simulink model "rlsest"  (Simulink 6.0)
settings: Solver=VariableStepDiscrete  SolverMode=SingleTasking  StartTime=0.0  StopTime=200  MaxStep=1  RelTol=1e-3  AbsTol=1e-6
StartFcn:
  | rlspps([],[],[],'reset',find_system(get_param(gcs,'Handle'),'LookUnderMasks','all','Tag','PPC'));
settings Model: Creator=The MathWorks Inc.  LastModifiedBy=batserve  ExtModeTrigMode=oneshot  ExtModeArmWhenConnect=off  ExtModeAutoUpdateStatusClock=off
settings DataIOCC: ExternalInput=[]  LimitDataPoints=off  SaveOutput=off  SaveTime=off
settings OptimizationCC: BooleanDataType=off
settings DebuggingCC: CheckExecutionContextPreStartOutputMsg=on  CheckExecutionContextRuntimeOutputMsg=on  SolverPrmCheckMsg=none  IntegerOverflowMsg=none
settings HardwareCC: TargetUnknown=on

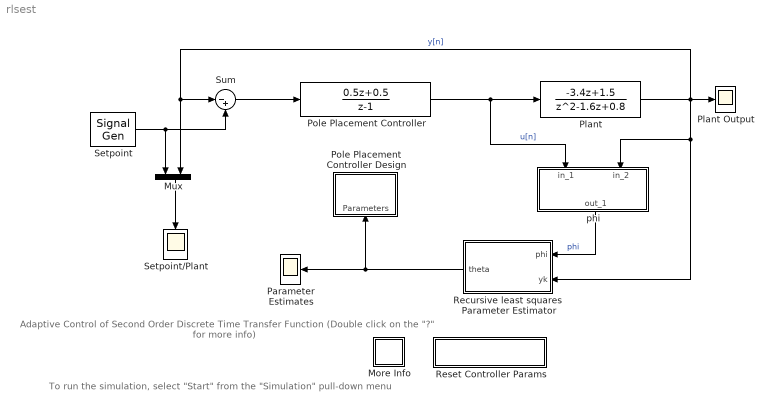
== system rlsest ==
  note: Adaptive Control of Second Order
      | Discrete Time Transfer Function
      | (Double click on the "?" for more info)
  note: To run the simulation, select "Start"
      | from the "Simulation" pull-down menu
  More Info : Subsystem  PropExecContextAcrossSSBoundary=on
      mask Display: disp('?')
  Mux : Mux  Orientation=down  Inputs=2
  Parameter Estimates : Scope
      settings: TickLabels=on  TimeRange=100.000000  DataFormat=Array
  Plant : DiscreteTransferFcn  Numerator=[-3.4 1.5]  Denominator=[1 -1.6 0.8]
  Plant Output : Scope
      settings: TickLabels=on  TimeRange=100.000000  DataFormat=Array
  Pole Placement Controller Design : Subsystem  Orientation=up  PropExecContextAcrossSSBoundary=on  mask(Pole Placement){@1=rlsest/Pole Placement Controller, @2=2, @3=poly([.6 .6 .6]), @4=10}
      mask prompts: @1 "Block name:"; @2 "Model order:"; @3 "Characteristic polynomial:"; @4 "Sample time:"
      mask help: Pole placement controller - installs new controller gains based upon a characteristic polynomial.
      mask init:
      | name=&1;order=@2;char_poly=@3;ts=@4;
      mask Help: Implements a pole placement design scheme for a discrete time controller.  Change the characteristic polynomial to see how the closed loop behavior changes.
      mask Display: disp('rlsppd')
  Pole Placement Controller : DiscreteTransferFcn  Tag=PPC  Numerator=[0.5 0.5]  Denominator=[1 -1]
  Recursive least squares  Parameter Estimator : Subsystem  Orientation=left  PropExecContextAcrossSSBoundary=on  mask(RLS Estimator){@1=2, @2=0.8, @3=1}
      mask prompts: @1 "Model Order:"; @2 "Forgetting Factor:"; @3 "Sample Time:"
      mask help: Hook input 1 to a state vector, and input 2 to the system output.
      mask init:
      | nstates = 2*@1;lambda=@2;ts=@3;
      mask Help: Implements a Recursive Least Squares parameter estimator. Mask and unmask this block to see how it works.
      mask Display: disp('RLS\nEstimator')
  Reset Controller Params : Subsystem  PropExecContextAcrossSSBoundary=on
      settings: OpenFcn=rlspps([],[],[],'reset',find_system(get_param(gcs,'Handle'),'LookUnderMasks','all','Tag','PPC'));
      mask Display: disp('Reset Controller')
  Setpoint : SignalGenerator  WaveForm=square  Amplitude=5.000000  Frequency=0.100000  Units=rad/sec
  Setpoint/Plant : Scope
      settings: Orientation=down  TickLabels=on  TimeRange=100.000000  DataFormat=Array
  Sum : Sum  Inputs=|-+  SaturateOnIntegerOverflow=on  InputSameDT=on
  phi : Subsystem  Orientation=down  PropExecContextAcrossSSBoundary=on  mask(State Generator){@1=2, @2=1}
      mask prompts: @1 "Model Order:"; @2 "Sample Time:"
      mask help: State Generator:
      mask init:
      | order = @1;ts = @2;
      mask Help: This block generates the state vector for use with the RLS parameter estimator.
      mask Display: disp('State\nGenerator')
  wires:
  Mux/1 -> Setpoint/Plant/1
  phi/1(out_1) -> Recursive least squares  Parameter Estimator/1(phi)  "phi"
  Pole Placement Controller/1 -> Plant/1, phi/1(in_1)  "u[n]"
  Sum/1 -> Pole Placement Controller/1
  Plant/1 -> Plant Output/1, Recursive least squares  Parameter Estimator/2(yk), phi/2(in_2), Mux/2, Sum/1  "y[n]"
  Recursive least squares  Parameter Estimator/1(theta) -> Pole Placement Controller Design/1(Parameters), Parameter Estimates/1
  Setpoint/1 -> Mux/1, Sum/2

== system rlsest/More Info ==
  note: Modify the parameters of the Plant during a simulation and observe
      | that the adaptive controller always maintains stability.
  note: This adaptive controller was implemented using the set_param
      | command in the M-file rlsppd. Unmask the other blocks
      | to see how they were implemented.
  note: This demonstration shows how an adaptive controller can
      | be designed and simulated.

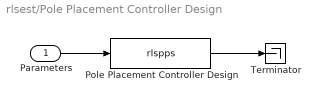
== system rlsest/Pole Placement Controller Design ==
  Parameters : Inport  Port=1  LatchInput=off
  Pole Placement Controller Design : S-Function  FunctionName=rlspps  Parameters=name,order,char_poly,ts
  Terminator : Terminator
  wires:
  Parameters/1 -> Pole Placement Controller Design/1
  Pole Placement Controller Design/1 -> Terminator/1

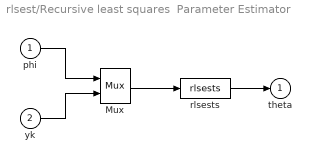
== system rlsest/Recursive least squares  Parameter Estimator ==
  phi : Inport  Port=1  LatchInput=off
  yk : Inport  Port=2  LatchInput=off
  Mux : Mux  Inputs=[nstates 1]
  rlsests : S-Function  FunctionName=rlsests  Parameters=nstates,lambda,ts
  theta : Outport  InitialOutput=0
  wires:
  yk/1 -> Mux/2
  rlsests/1 -> theta/1
  phi/1 -> Mux/1
  Mux/1 -> rlsests/1

== system rlsest/Reset Controller Params ==

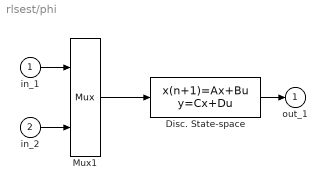
== system rlsest/phi ==
  in_1 : Inport  Port=1  LatchInput=off
  in_2 : Inport  Port=2  LatchInput=off
  Disc. State-space : DiscreteStateSpace  A=[zeros(1,2*order);eye(order-1,2*order);zeros(1,2*order);zeros(order-1,order),eye(order-1,order)]  B=[1, zeros(1,2*order-1);zeros(1,order),-1,zeros(1,order-1)]'  C=eye(2*order)  D=[zeros(2*order,order)]  SampleTime=ts
  Mux1 : Mux  Inputs=[1 1]
  out_1 : Outport  InitialOutput=0
  wires:
  Mux1/1 -> Disc. State-space/1
  in_1/1 -> Mux1/1
  Disc. State-space/1 -> out_1/1
  in_2/1 -> Mux1/2
